simulink model "exercise2"  (R2024b)
settings: Solver=VariableStepAuto  StartTime=0.0  StopTime=10.0  RelTol=1e-3
settings Model: Creator=sadra  LastModifiedBy=sadra

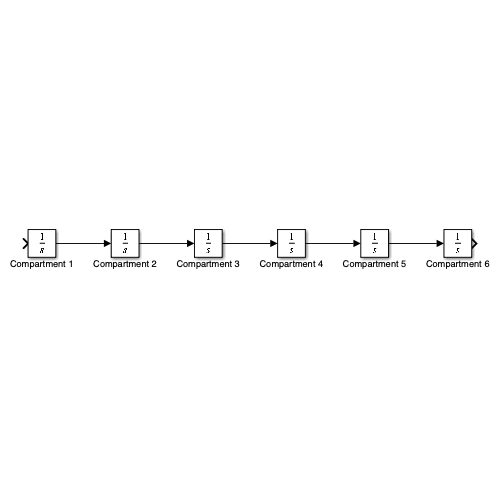
[thumbnail: Simulink's stored preview of the top-level diagram]
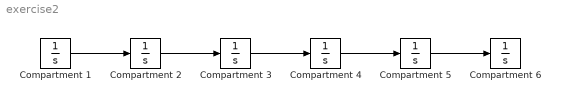
== system exercise2 ==
  Compartment {1..6} (6 alike) : Integrator
  wires:
  Compartment 2/1 -> Compartment 3/1
  Compartment 3/1 -> Compartment 4/1
  Compartment 4/1 -> Compartment 5/1
  Compartment 5/1 -> Compartment 6/1
  Compartment 1/1 -> Compartment 2/1
